simulink model "propagatorN1"  (R2019b)
settings: Solver=ode113  StartTime=0.0  StopTime=86400  MaxStep=0.05  MinStep=1e-4  RelTol=1e-3  AbsTol=1e-13
model workspace (MAT data in the model file):
  mi = 1
undefined symbols (not defined in the file or in its folder): ParAltimeter, ParBody, ParCamera, ParEphemerides, ParRadio, ParSpacecraft
settings Model: Creator=tomma  LastModifiedBy=antoniogenova

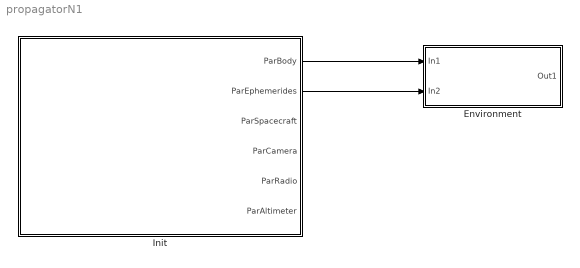
== system propagatorN1 ==
  Environment : Subsystem
  "Init " : Subsystem
  wires:
  "Init "/1(ParBody) -> Environment/1(In1)
  "Init "/2(ParEphemerides) -> Environment/2(In2)

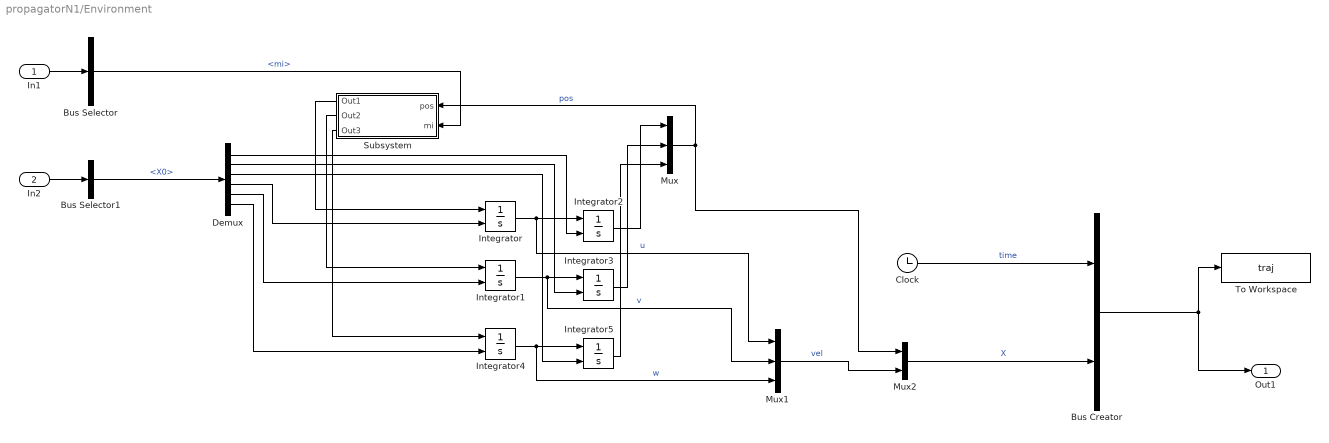
== system propagatorN1/Environment ==
  In1 : Inport
  In2 : Inport  Port=2
  Bus Creator : BusCreator  Inputs=2
  Bus Selector : BusSelector  OutputSignals=ParBody_Bus.mi
  Bus Selector1 : BusSelector  OutputSignals=ParEphemerides_Bus.X0
  Clock : Clock
  Demux : Demux  Outputs=6
  Integrator{,1..5} (6 alike) : Integrator  InitialConditionSource=external  ContinuousStateAttributes="\"\""
  Mux : Mux  Inputs=3
  Mux1 : Mux  Inputs=3
  Mux2 : Mux  Inputs=2
  Subsystem : Subsystem
  To Workspace : ToWorkspace  VariableName=traj  SaveFormat=Timeseries  SampleTime=-1
  Out1 : Outport
  wires:
  Integrator1/1 -> Mux1/2, Integrator3/1  "v"
  Clock/1 -> Bus Creator/1  "time"
  Bus Creator/1 -> Out1/1, To Workspace/1
  Integrator4/1 -> Mux1/3, Integrator5/1  "w"
  Subsystem/3(Out3) -> Integrator4/1
  Integrator2/1 -> Mux/1
  Demux/2 -> Integrator3/2
  Demux/3 -> Integrator5/2
  Mux2/1 -> Bus Creator/2  "X"
  Subsystem/2(Out2) -> Integrator1/1
  Integrator3/1 -> Mux/2
  Mux/1 -> Mux2/1, Subsystem/1(pos)  "pos"
  Integrator5/1 -> Mux/3
  Demux/6 -> Integrator4/2
  Demux/1 -> Integrator2/2
  Integrator/1 -> Mux1/1, Integrator2/1  "u"
  Mux1/1 -> Mux2/2  "vel"
  Subsystem/1(Out1) -> Integrator/1
  Demux/4 -> Integrator/2
  Demux/5 -> Integrator1/2
  Bus Selector1/1 -> Demux/1  "<X0>"
  In1/1 -> Bus Selector/1
  In2/1 -> Bus Selector1/1
  Bus Selector/1 -> Subsystem/2(mi)  "<mi>"

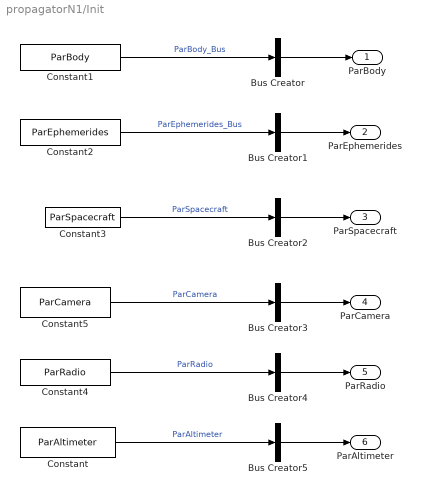
== system propagatorN1/Init  ==
  Bus Creator{,1..5} (6 alike) : BusCreator  Inputs=1
  Constant : Constant  Value=ParAltimeter  OutDataTypeStr=Bus: ParAltimeter_Bus
  Constant1 : Constant  Value=ParBody  OutDataTypeStr=Bus: ParBody_Bus
  Constant2 : Constant  Value=ParEphemerides  OutDataTypeStr=Bus: ParEphemerides_Bus
  Constant3 : Constant  Value=ParSpacecraft  OutDataTypeStr=Bus: ParSpacecraft_Bus
  Constant4 : Constant  Value=ParRadio  OutDataTypeStr=Bus: ParRadio_Bus
  Constant5 : Constant  Value=ParCamera  OutDataTypeStr=Bus: ParCamera_Bus
  ParBody : Outport
  ParEphemerides : Outport  Port=2
  ParSpacecraft : Outport  Port=3
  ParCamera : Outport  Port=4
  ParRadio : Outport  Port=5
  ParAltimeter : Outport  Port=6
  wires:
  Constant/1 -> Bus Creator5/1  "ParAltimeter"
  Constant5/1 -> Bus Creator3/1  "ParCamera"
  Constant4/1 -> Bus Creator4/1  "ParRadio"
  Constant1/1 -> Bus Creator/1  "ParBody_Bus"
  Constant2/1 -> Bus Creator1/1  "ParEphemerides_Bus"
  Constant3/1 -> Bus Creator2/1  "ParSpacecraft"
  Bus Creator/1 -> ParBody/1
  Bus Creator1/1 -> ParEphemerides/1
  Bus Creator2/1 -> ParSpacecraft/1
  Bus Creator3/1 -> ParCamera/1
  Bus Creator4/1 -> ParRadio/1
  Bus Creator5/1 -> ParAltimeter/1

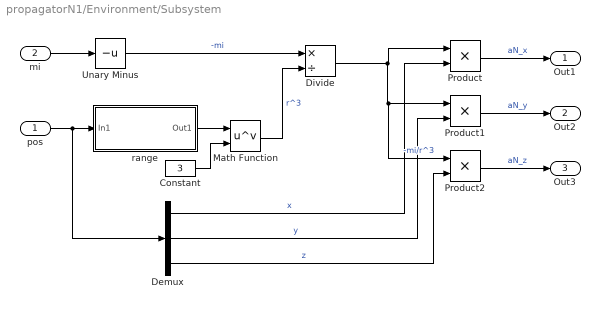
== system propagatorN1/Environment/Subsystem ==
  pos : Inport
  mi : Inport  Port=2
  Constant : Constant  Value=3
  Demux : Demux  Outputs=3
  Divide : Product  Inputs=*/
  Math Function : Math  Operator=pow  SignedPower=off  SaturateOnIntegerOverflow=on
  Product : Product
  Product1 : Product
  Product2 : Product
  Unary Minus : UnaryMinus
  range : Subsystem
  Out1 : Outport
  Out2 : Outport  Port=2
  Out3 : Outport  Port=3
  wires:
  pos/1 -> Demux/1, range/1(In1)
  mi/1 -> Unary Minus/1
  Unary Minus/1 -> Divide/1  "-mi"
  Constant/1 -> Math Function/2
  range/1(Out1) -> Math Function/1
  Math Function/1 -> Divide/2  "r^3"
  Divide/1 -> Product2/1, Product1/1, Product/1  "-mi/r^3"
  Demux/1 -> Product/2  "x"
  Demux/2 -> Product1/2  "y"
  Demux/3 -> Product2/2  "z"
  Product/1 -> Out1/1  "aN_x"
  Product1/1 -> Out2/1  "aN_y"
  Product2/1 -> Out3/1  "aN_z"

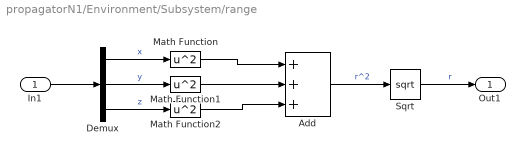
== system propagatorN1/Environment/Subsystem/range ==
  In1 : Inport
  Add : Sum  Inputs=+++
  Demux : Demux  Outputs=3
  Math Function : Math  Operator=square  SignedPower=off  SaturateOnIntegerOverflow=on
  Math Function1 : Math  Operator=square  SignedPower=off  SaturateOnIntegerOverflow=on
  Math Function2 : Math  Operator=square  SignedPower=off  SaturateOnIntegerOverflow=on
  Sqrt : Sqrt  SaturateOnIntegerOverflow=on
  Out1 : Outport
  wires:
  In1/1 -> Demux/1
  Demux/1 -> Math Function/1  "x"
  Demux/2 -> Math Function1/1  "y"
  Demux/3 -> Math Function2/1  "z"
  Math Function/1 -> Add/1
  Math Function1/1 -> Add/2
  Math Function2/1 -> Add/3
  Add/1 -> Sqrt/1  "r^2"
  Sqrt/1 -> Out1/1  "r"
